simulink model "TST_CrCtl_Governor"  (R2016b)
settings: Solver=FixedStepDiscrete  StartTime=0.0  StopTime=simTime  FixedStep=sampleTime  RelTol=1e-3
values from neighbouring files (symbols this model uses):
  testCase = 1    [initTST_CrCtl_Governor_001.m]    (also in initTST_CrCtl_Governor_002.m = 2; initTST_CrCtl_Governor_003.m = 3; initTST_CrCtl_Governor_004.m = 4; initTST_CrCtl_Governor_005.m = 5)
libraries: simulink x144, UnitTest_Lib x110
(part 6 of 7)

== system TST_CrCtl_Governor/simulationInput/testSignals_R008 ==
  BC : BusCreator  Inputs=54
  spec_APP_r : FromWorkspace  VariableName=testSig_APP_r  Interpolate=off  OutputAfterFinalValue=Holding final value
  spec_AccPed_trqDes : FromWorkspace  VariableName=testSig_AccPed_trqDes  Interpolate=off  OutputAfterFinalValue=Holding final value
  spec_CoETS_trqNTCActvOff : FromWorkspace  VariableName=testSig_CoETS_trqNTCActvOff  Interpolate=off  OutputAfterFinalValue=Holding final value
  spec_CoETS_trqNTCActvOn : FromWorkspace  VariableName=testSig_CoETS_trqNTCActvOn  Interpolate=off  OutputAfterFinalValue=Holding final value
  spec_CoETS_trqUnFltLtd : FromWorkspace  VariableName=testSig_CoETS_trqUnFltLtd  Interpolate=off  OutputAfterFinalValue=Holding final value
  spec_CoVMD_trqLLim : FromWorkspace  VariableName=testSig_CoVMD_trqLLim  Interpolate=off  OutputAfterFinalValue=Holding final value
  spec_CoVeh_trqAcs : FromWorkspace  VariableName=testSig_CoVeh_trqAcs  Interpolate=off  OutputAfterFinalValue=Holding final value
  spec_CoVeh_trqPrpLimErr : FromWorkspace  VariableName=testSig_CoVeh_trqPrpLimErr  Interpolate=off  OutputAfterFinalValue=Holding final value
  spec_CrCtl_aAccThres : FromWorkspace  VariableName=testSig_CrCtl_aAccThres  Interpolate=off  OutputAfterFinalValue=Holding final value
  spec_CrCtl_aDeclThres : FromWorkspace  VariableName=testSig_CrCtl_aDeclThres  Interpolate=off  OutputAfterFinalValue=Holding final value
  spec_CrCtl_rTraV2NBeg : FromWorkspace  VariableName=testSig_CrCtl_rTraV2NBeg  Interpolate=off  OutputAfterFinalValue=Holding final value
  spec_CrCtl_st : FromWorkspace  VariableName=testSig_CrCtl_st  Interpolate=off  OutputAfterFinalValue=Holding final value
  spec_CrCtl_stGvnr : FromWorkspace  VariableName=testSig_CrCtl_stGvnr  Interpolate=off  OutputAfterFinalValue=Holding final value
  spec_CrCtl_stLck : FromWorkspace  VariableName=testSig_CrCtl_stLck  Interpolate=off  OutputAfterFinalValue=Holding final value
  spec_CrCtl_stOpFunc : FromWorkspace  VariableName=testSig_CrCtl_stOpFunc  Interpolate=off  OutputAfterFinalValue=Holding final value
  spec_CrCtl_stPtd : FromWorkspace  VariableName=testSig_CrCtl_stPtd  Interpolate=off  OutputAfterFinalValue=Holding final value
  spec_CrCtl_stReq : FromWorkspace  VariableName=testSig_CrCtl_stReq  Interpolate=off  OutputAfterFinalValue=Holding final value
  spec_CrCtl_stShOff : FromWorkspace  VariableName=testSig_CrCtl_stShOff  Interpolate=off  OutputAfterFinalValue=Holding final value
  spec_CrCtl_stSub : FromWorkspace  VariableName=testSig_CrCtl_stSub  Interpolate=off  OutputAfterFinalValue=Holding final value
  spec_CrCtl_stSubGvnr : FromWorkspace  VariableName=testSig_CrCtl_stSubGvnr  Interpolate=off  OutputAfterFinalValue=Holding final value
  spec_CrCtl_stSuspAct : FromWorkspace  VariableName=testSig_CrCtl_stSuspAct  Interpolate=off  OutputAfterFinalValue=Holding final value
  spec_CrCtl_stSuspRamp : FromWorkspace  VariableName=testSig_CrCtl_stSuspRamp  Interpolate=off  OutputAfterFinalValue=Holding final value
  spec_CrCtl_stVDirChng : FromWorkspace  VariableName=testSig_CrCtl_stVDirChng  Interpolate=off  OutputAfterFinalValue=Holding final value
  spec_CrCtl_stvHysEngBrkReq : FromWorkspace  VariableName=testSig_CrCtl_stvHysEngBrkReq  Interpolate=off  OutputAfterFinalValue=Holding final value
  spec_CrCtl_trqLead : FromWorkspace  VariableName=testSig_CrCtl_trqLead  Interpolate=off  OutputAfterFinalValue=Holding final value
  spec_CrCtl_trqLimAct : FromWorkspace  VariableName=testSig_CrCtl_trqLimAct  Interpolate=off  OutputAfterFinalValue=Holding final value
  spec_CrCtl_trqMin : FromWorkspace  VariableName=testSig_CrCtl_trqMin  Interpolate=off  OutputAfterFinalValue=Holding final value
  spec_CrCtl_trqReq : FromWorkspace  VariableName=testSig_CrCtl_trqReq  Interpolate=off  OutputAfterFinalValue=Holding final value
  spec_CrCtl_trqReqOld : FromWorkspace  VariableName=testSig_CrCtl_trqReqOld  Interpolate=off  OutputAfterFinalValue=Holding final value
  spec_CrCtl_vDes : FromWorkspace  VariableName=testSig_CrCtl_vDes  Interpolate=off  OutputAfterFinalValue=Holding final value
  spec_CrCtl_vDesAct : FromWorkspace  VariableName=testSig_CrCtl_vDesAct  Interpolate=off  OutputAfterFinalValue=Holding final value
  spec_CrCtl_vDesActOld : FromWorkspace  VariableName=testSig_CrCtl_vDesActOld  Interpolate=off  OutputAfterFinalValue=Holding final value
  spec_CrCtl_vMax : FromWorkspace  VariableName=testSig_CrCtl_vMax  Interpolate=off  OutputAfterFinalValue=Holding final value
  spec_CrCtl_vMaxDvtAcc : FromWorkspace  VariableName=testSig_CrCtl_vMaxDvtAcc  Interpolate=off  OutputAfterFinalValue=Holding final value
  spec_CrCtl_vMaxDvtDecl : FromWorkspace  VariableName=testSig_CrCtl_vMaxDvtDecl  Interpolate=off  OutputAfterFinalValue=Holding final value
  spec_CrCtl_vMin : FromWorkspace  VariableName=testSig_CrCtl_vMin  Interpolate=off  OutputAfterFinalValue=Holding final value
  spec_EBrk_stPreSelMode : FromWorkspace  VariableName=testSig_EBrk_stPreSelMode  Interpolate=off  OutputAfterFinalValue=Holding final value
  spec_EngDem_trqInrLim : FromWorkspace  VariableName=testSig_EngDem_trqInrLim  Interpolate=off  OutputAfterFinalValue=Holding final value
  spec_GlbDa_aXFlt : FromWorkspace  VariableName=testSig_GlbDa_aXFlt  Interpolate=off  OutputAfterFinalValue=Holding final value
  spec_GlbDa_vXFlt : FromWorkspace  VariableName=testSig_GlbDa_vXFlt  Interpolate=off  OutputAfterFinalValue=Holding final value
  spec_InjSys_trqLim : FromWorkspace  VariableName=testSig_InjSys_trqLim  Interpolate=off  OutputAfterFinalValue=Holding final value
  spec_PT_rTraV2N : FromWorkspace  VariableName=testSig_PT_rTraV2N  Interpolate=off  OutputAfterFinalValue=Holding final value
  spec_PT_rTrq : FromWorkspace  VariableName=testSig_PT_rTrq  Interpolate=off  OutputAfterFinalValue=Holding final value
  spec_PT_trqLos : FromWorkspace  VariableName=testSig_PT_trqLos  Interpolate=off  OutputAfterFinalValue=Holding final value
  spec_PT_trqWhl : FromWorkspace  VariableName=testSig_PT_trqWhl  Interpolate=off  OutputAfterFinalValue=Holding final value
  spec_PT_trqWhlMinEng : FromWorkspace  VariableName=testSig_PT_trqWhlMinEng  Interpolate=off  OutputAfterFinalValue=Holding final value
  spec_PT_trqWhlMinEngBrk : FromWorkspace  VariableName=testSig_PT_trqWhlMinEngBrk  Interpolate=off  OutputAfterFinalValue=Holding final value
  spec_RngMod_trqMin : FromWorkspace  VariableName=testSig_RngMod_trqMin  Interpolate=off  OutputAfterFinalValue=Holding final value
  spec_Tra_numGear : FromWorkspace  VariableName=testSig_Tra_numGear  Interpolate=off  OutputAfterFinalValue=Holding final value
  spec_VMD_trqDes : FromWorkspace  VariableName=testSig_VMD_trqDes  Interpolate=off  OutputAfterFinalValue=Holding final value
  spec_VMSAdjBtn_st : FromWorkspace  VariableName=testSig_VMSAdjBtn_st  Interpolate=off  OutputAfterFinalValue=Holding final value
  spec_VMSLmtSwt_st : FromWorkspace  VariableName=testSig_VMSLmtSwt_st  Interpolate=off  OutputAfterFinalValue=Holding final value
  spec_VehMot_rTrqDfftl : FromWorkspace  VariableName=testSig_VehMot_rTrqDfftl  Interpolate=off  OutputAfterFinalValue=Holding final value
  spec_WESDem_stCurr : FromWorkspace  VariableName=testSig_WESDem_stCurr  Interpolate=off  OutputAfterFinalValue=Holding final value
  testSignals : Outport
  wires:
  BC/1 -> testSignals/1
  spec_AccPed_trqDes/1 -> BC/1  "testSig_AccPed_trqDes"
  spec_APP_r/1 -> BC/2  "testSig_APP_r"
  spec_CoETS_trqNTCActvOff/1 -> BC/3  "testSig_CoETS_trqNTCActvOff"
  spec_CoETS_trqNTCActvOn/1 -> BC/4  "testSig_CoETS_trqNTCActvOn"
  spec_CoETS_trqUnFltLtd/1 -> BC/5  "testSig_CoETS_trqUnFltLtd"
  spec_CoVeh_trqAcs/1 -> BC/6  "testSig_CoVeh_trqAcs"
  spec_CoVeh_trqPrpLimErr/1 -> BC/7  "testSig_CoVeh_trqPrpLimErr"
  spec_CoVMD_trqLLim/1 -> BC/8  "testSig_CoVMD_trqLLim"
  spec_CrCtl_aAccThres/1 -> BC/9  "testSig_CrCtl_aAccThres"
  spec_CrCtl_aDeclThres/1 -> BC/10  "testSig_CrCtl_aDeclThres"
  spec_CrCtl_st/1 -> BC/11  "testSig_CrCtl_st"
  spec_CrCtl_stGvnr/1 -> BC/12  "testSig_CrCtl_stGvnr"
  spec_CrCtl_stLck/1 -> BC/13  "testSig_CrCtl_stLck"
  spec_CrCtl_stShOff/1 -> BC/14  "testSig_CrCtl_stShOff"
  spec_CrCtl_stSub/1 -> BC/15  "testSig_CrCtl_stSub"
  spec_CrCtl_stSubGvnr/1 -> BC/16  "testSig_CrCtl_stSubGvnr"
  spec_CrCtl_stSuspAct/1 -> BC/17  "testSig_CrCtl_stSuspAct"
  spec_CrCtl_stVDirChng/1 -> BC/18  "testSig_CrCtl_stVDirChng"
  spec_CrCtl_vDes/1 -> BC/19  "testSig_CrCtl_vDes"
  spec_CrCtl_vDesAct/1 -> BC/20  "testSig_CrCtl_vDesAct"
  spec_CrCtl_vDesActOld/1 -> BC/21  "testSig_CrCtl_vDesActOld"
  spec_CrCtl_vMaxDvtAcc/1 -> BC/22  "testSig_CrCtl_vMaxDvtAcc"
  spec_CrCtl_vMaxDvtDecl/1 -> BC/23  "testSig_CrCtl_vMaxDvtDecl"
  spec_CrCtl_vMin/1 -> BC/24  "testSig_CrCtl_vMin"
  spec_EBrk_stPreSelMode/1 -> BC/25  "testSig_EBrk_stPreSelMode"
  spec_EngDem_trqInrLim/1 -> BC/26  "testSig_EngDem_trqInrLim"
  spec_GlbDa_aXFlt/1 -> BC/27  "testSig_GlbDa_aXFlt"
  spec_GlbDa_vXFlt/1 -> BC/28  "testSig_GlbDa_vXFlt"
  spec_InjSys_trqLim/1 -> BC/29  "testSig_InjSys_trqLim"
  spec_PT_rTraV2N/1 -> BC/30  "testSig_PT_rTraV2N"
  spec_PT_rTrq/1 -> BC/31  "testSig_PT_rTrq"
  spec_PT_trqLos/1 -> BC/32  "testSig_PT_trqLos"
  spec_PT_trqWhl/1 -> BC/33  "testSig_PT_trqWhl"
  spec_PT_trqWhlMinEng/1 -> BC/34  "testSig_PT_trqWhlMinEng"
  spec_PT_trqWhlMinEngBrk/1 -> BC/35  "testSig_PT_trqWhlMinEngBrk"
  spec_RngMod_trqMin/1 -> BC/36  "testSig_RngMod_trqMin"
  spec_Tra_numGear/1 -> BC/37  "testSig_Tra_numGear"
  spec_VehMot_rTrqDfftl/1 -> BC/38  "testSig_VehMot_rTrqDfftl"
  spec_VMD_trqDes/1 -> BC/39  "testSig_VMD_trqDes"
  spec_VMSAdjBtn_st/1 -> BC/40  "testSig_VMSAdjBtn_st"
  spec_VMSLmtSwt_st/1 -> BC/41  "testSig_VMSLmtSwt_st"
  spec_WESDem_stCurr/1 -> BC/42  "testSig_WESDem_stCurr"
  spec_CrCtl_rTraV2NBeg/1 -> BC/43  "testSig_CrCtl_rTraV2NBeg"
  spec_CrCtl_stOpFunc/1 -> BC/44  "testSig_CrCtl_stOpFunc"
  spec_CrCtl_stPtd/1 -> BC/45  "testSig_CrCtl_stPtd"
  spec_CrCtl_stReq/1 -> BC/46  "testSig_CrCtl_stReq"
  spec_CrCtl_stSuspRamp/1 -> BC/47  "testSig_CrCtl_stSuspRamp"
  spec_CrCtl_stvHysEngBrkReq/1 -> BC/48  "testSig_CrCtl_stvHysEngBrkReq"
  spec_CrCtl_trqLead/1 -> BC/49  "testSig_CrCtl_trqLead"
  spec_CrCtl_trqLimAct/1 -> BC/50  "testSig_CrCtl_trqLimAct"
  spec_CrCtl_trqMin/1 -> BC/51  "testSig_CrCtl_trqMin"
  spec_CrCtl_trqReq/1 -> BC/52  "testSig_CrCtl_trqReq"
  spec_CrCtl_trqReqOld/1 -> BC/53  "testSig_CrCtl_trqReqOld"
  spec_CrCtl_vMax/1 -> BC/54  "testSig_CrCtl_vMax"

== system TST_CrCtl_Governor/simulationInput/testSignals_R009 ==
  BC : BusCreator  Inputs=54
  spec_APP_r : FromWorkspace  VariableName=testSig_APP_r  Interpolate=off  OutputAfterFinalValue=Holding final value
  spec_AccPed_trqDes : FromWorkspace  VariableName=testSig_AccPed_trqDes  Interpolate=off  OutputAfterFinalValue=Holding final value
  spec_CoETS_trqNTCActvOff : FromWorkspace  VariableName=testSig_CoETS_trqNTCActvOff  Interpolate=off  OutputAfterFinalValue=Holding final value
  spec_CoETS_trqNTCActvOn : FromWorkspace  VariableName=testSig_CoETS_trqNTCActvOn  Interpolate=off  OutputAfterFinalValue=Holding final value
  spec_CoETS_trqUnFltLtd : FromWorkspace  VariableName=testSig_CoETS_trqUnFltLtd  Interpolate=off  OutputAfterFinalValue=Holding final value
  spec_CoVMD_trqLLim : FromWorkspace  VariableName=testSig_CoVMD_trqLLim  Interpolate=off  OutputAfterFinalValue=Holding final value
  spec_CoVeh_trqAcs : FromWorkspace  VariableName=testSig_CoVeh_trqAcs  Interpolate=off  OutputAfterFinalValue=Holding final value
  spec_CoVeh_trqPrpLimErr : FromWorkspace  VariableName=testSig_CoVeh_trqPrpLimErr  Interpolate=off  OutputAfterFinalValue=Holding final value
  spec_CrCtl_aAccThres : FromWorkspace  VariableName=testSig_CrCtl_aAccThres  Interpolate=off  OutputAfterFinalValue=Holding final value
  spec_CrCtl_aDeclThres : FromWorkspace  VariableName=testSig_CrCtl_aDeclThres  Interpolate=off  OutputAfterFinalValue=Holding final value
  spec_CrCtl_rTraV2NBeg : FromWorkspace  VariableName=testSig_CrCtl_rTraV2NBeg  Interpolate=off  OutputAfterFinalValue=Holding final value
  spec_CrCtl_st : FromWorkspace  VariableName=testSig_CrCtl_st  Interpolate=off  OutputAfterFinalValue=Holding final value
  spec_CrCtl_stGvnr : FromWorkspace  VariableName=testSig_CrCtl_stGvnr  Interpolate=off  OutputAfterFinalValue=Holding final value
  spec_CrCtl_stLck : FromWorkspace  VariableName=testSig_CrCtl_stLck  Interpolate=off  OutputAfterFinalValue=Holding final value
  spec_CrCtl_stOpFunc : FromWorkspace  VariableName=testSig_CrCtl_stOpFunc  Interpolate=off  OutputAfterFinalValue=Holding final value
  spec_CrCtl_stPtd : FromWorkspace  VariableName=testSig_CrCtl_stPtd  Interpolate=off  OutputAfterFinalValue=Holding final value
  spec_CrCtl_stReq : FromWorkspace  VariableName=testSig_CrCtl_stReq  Interpolate=off  OutputAfterFinalValue=Holding final value
  spec_CrCtl_stShOff : FromWorkspace  VariableName=testSig_CrCtl_stShOff  Interpolate=off  OutputAfterFinalValue=Holding final value
  spec_CrCtl_stSub : FromWorkspace  VariableName=testSig_CrCtl_stSub  Interpolate=off  OutputAfterFinalValue=Holding final value
  spec_CrCtl_stSubGvnr : FromWorkspace  VariableName=testSig_CrCtl_stSubGvnr  Interpolate=off  OutputAfterFinalValue=Holding final value
  spec_CrCtl_stSuspAct : FromWorkspace  VariableName=testSig_CrCtl_stSuspAct  Interpolate=off  OutputAfterFinalValue=Holding final value
  spec_CrCtl_stSuspRamp : FromWorkspace  VariableName=testSig_CrCtl_stSuspRamp  Interpolate=off  OutputAfterFinalValue=Holding final value
  spec_CrCtl_stVDirChng : FromWorkspace  VariableName=testSig_CrCtl_stVDirChng  Interpolate=off  OutputAfterFinalValue=Holding final value
  spec_CrCtl_stvHysEngBrkReq : FromWorkspace  VariableName=testSig_CrCtl_stvHysEngBrkReq  Interpolate=off  OutputAfterFinalValue=Holding final value
  spec_CrCtl_trqLead : FromWorkspace  VariableName=testSig_CrCtl_trqLead  Interpolate=off  OutputAfterFinalValue=Holding final value
  spec_CrCtl_trqLimAct : FromWorkspace  VariableName=testSig_CrCtl_trqLimAct  Interpolate=off  OutputAfterFinalValue=Holding final value
  spec_CrCtl_trqMin : FromWorkspace  VariableName=testSig_CrCtl_trqMin  Interpolate=off  OutputAfterFinalValue=Holding final value
  spec_CrCtl_trqReq : FromWorkspace  VariableName=testSig_CrCtl_trqReq  Interpolate=off  OutputAfterFinalValue=Holding final value
  spec_CrCtl_trqReqOld : FromWorkspace  VariableName=testSig_CrCtl_trqReqOld  Interpolate=off  OutputAfterFinalValue=Holding final value
  spec_CrCtl_vDes : FromWorkspace  VariableName=testSig_CrCtl_vDes  Interpolate=off  OutputAfterFinalValue=Holding final value
  spec_CrCtl_vDesAct : FromWorkspace  VariableName=testSig_CrCtl_vDesAct  Interpolate=off  OutputAfterFinalValue=Holding final value
  spec_CrCtl_vDesActOld : FromWorkspace  VariableName=testSig_CrCtl_vDesActOld  Interpolate=off  OutputAfterFinalValue=Holding final value
  spec_CrCtl_vMax : FromWorkspace  VariableName=testSig_CrCtl_vMax  Interpolate=off  OutputAfterFinalValue=Holding final value
  spec_CrCtl_vMaxDvtAcc : FromWorkspace  VariableName=testSig_CrCtl_vMaxDvtAcc  Interpolate=off  OutputAfterFinalValue=Holding final value
  spec_CrCtl_vMaxDvtDecl : FromWorkspace  VariableName=testSig_CrCtl_vMaxDvtDecl  Interpolate=off  OutputAfterFinalValue=Holding final value
  spec_CrCtl_vMin : FromWorkspace  VariableName=testSig_CrCtl_vMin  Interpolate=off  OutputAfterFinalValue=Holding final value
  spec_EBrk_stPreSelMode : FromWorkspace  VariableName=testSig_EBrk_stPreSelMode  Interpolate=off  OutputAfterFinalValue=Holding final value
  spec_EngDem_trqInrLim : FromWorkspace  VariableName=testSig_EngDem_trqInrLim  Interpolate=off  OutputAfterFinalValue=Holding final value
  spec_GlbDa_aXFlt : FromWorkspace  VariableName=testSig_GlbDa_aXFlt  Interpolate=off  OutputAfterFinalValue=Holding final value
  spec_GlbDa_vXFlt : FromWorkspace  VariableName=testSig_GlbDa_vXFlt  Interpolate=off  OutputAfterFinalValue=Holding final value
  spec_InjSys_trqLim : FromWorkspace  VariableName=testSig_InjSys_trqLim  Interpolate=off  OutputAfterFinalValue=Holding final value
  spec_PT_rTraV2N : FromWorkspace  VariableName=testSig_PT_rTraV2N  Interpolate=off  OutputAfterFinalValue=Holding final value
  spec_PT_rTrq : FromWorkspace  VariableName=testSig_PT_rTrq  Interpolate=off  OutputAfterFinalValue=Holding final value
  spec_PT_trqLos : FromWorkspace  VariableName=testSig_PT_trqLos  Interpolate=off  OutputAfterFinalValue=Holding final value
  spec_PT_trqWhl : FromWorkspace  VariableName=testSig_PT_trqWhl  Interpolate=off  OutputAfterFinalValue=Holding final value
  spec_PT_trqWhlMinEng : FromWorkspace  VariableName=testSig_PT_trqWhlMinEng  Interpolate=off  OutputAfterFinalValue=Holding final value
  spec_PT_trqWhlMinEngBrk : FromWorkspace  VariableName=testSig_PT_trqWhlMinEngBrk  Interpolate=off  OutputAfterFinalValue=Holding final value
  spec_RngMod_trqMin : FromWorkspace  VariableName=testSig_RngMod_trqMin  Interpolate=off  OutputAfterFinalValue=Holding final value
  spec_Tra_numGear : FromWorkspace  VariableName=testSig_Tra_numGear  Interpolate=off  OutputAfterFinalValue=Holding final value
  spec_VMD_trqDes : FromWorkspace  VariableName=testSig_VMD_trqDes  Interpolate=off  OutputAfterFinalValue=Holding final value
  spec_VMSAdjBtn_st : FromWorkspace  VariableName=testSig_VMSAdjBtn_st  Interpolate=off  OutputAfterFinalValue=Holding final value
  spec_VMSLmtSwt_st : FromWorkspace  VariableName=testSig_VMSLmtSwt_st  Interpolate=off  OutputAfterFinalValue=Holding final value
  spec_VehMot_rTrqDfftl : FromWorkspace  VariableName=testSig_VehMot_rTrqDfftl  Interpolate=off  OutputAfterFinalValue=Holding final value
  spec_WESDem_stCurr : FromWorkspace  VariableName=testSig_WESDem_stCurr  Interpolate=off  OutputAfterFinalValue=Holding final value
  testSignals : Outport
  wires:
  BC/1 -> testSignals/1
  spec_AccPed_trqDes/1 -> BC/1  "testSig_AccPed_trqDes"
  spec_APP_r/1 -> BC/2  "testSig_APP_r"
  spec_CoETS_trqNTCActvOff/1 -> BC/3  "testSig_CoETS_trqNTCActvOff"
  spec_CoETS_trqNTCActvOn/1 -> BC/4  "testSig_CoETS_trqNTCActvOn"
  spec_CoETS_trqUnFltLtd/1 -> BC/5  "testSig_CoETS_trqUnFltLtd"
  spec_CoVeh_trqAcs/1 -> BC/6  "testSig_CoVeh_trqAcs"
  spec_CoVeh_trqPrpLimErr/1 -> BC/7  "testSig_CoVeh_trqPrpLimErr"
  spec_CoVMD_trqLLim/1 -> BC/8  "testSig_CoVMD_trqLLim"
  spec_CrCtl_aAccThres/1 -> BC/9  "testSig_CrCtl_aAccThres"
  spec_CrCtl_aDeclThres/1 -> BC/10  "testSig_CrCtl_aDeclThres"
  spec_CrCtl_st/1 -> BC/11  "testSig_CrCtl_st"
  spec_CrCtl_stGvnr/1 -> BC/12  "testSig_CrCtl_stGvnr"
  spec_CrCtl_stLck/1 -> BC/13  "testSig_CrCtl_stLck"
  spec_CrCtl_stShOff/1 -> BC/14  "testSig_CrCtl_stShOff"
  spec_CrCtl_stSub/1 -> BC/15  "testSig_CrCtl_stSub"
  spec_CrCtl_stSubGvnr/1 -> BC/16  "testSig_CrCtl_stSubGvnr"
  spec_CrCtl_stSuspAct/1 -> BC/17  "testSig_CrCtl_stSuspAct"
  spec_CrCtl_stVDirChng/1 -> BC/18  "testSig_CrCtl_stVDirChng"
  spec_CrCtl_vDes/1 -> BC/19  "testSig_CrCtl_vDes"
  spec_CrCtl_vDesAct/1 -> BC/20  "testSig_CrCtl_vDesAct"
  spec_CrCtl_vDesActOld/1 -> BC/21  "testSig_CrCtl_vDesActOld"
  spec_CrCtl_vMaxDvtAcc/1 -> BC/22  "testSig_CrCtl_vMaxDvtAcc"
  spec_CrCtl_vMaxDvtDecl/1 -> BC/23  "testSig_CrCtl_vMaxDvtDecl"
  spec_CrCtl_vMin/1 -> BC/24  "testSig_CrCtl_vMin"
  spec_EBrk_stPreSelMode/1 -> BC/25  "testSig_EBrk_stPreSelMode"
  spec_EngDem_trqInrLim/1 -> BC/26  "testSig_EngDem_trqInrLim"
  spec_GlbDa_aXFlt/1 -> BC/27  "testSig_GlbDa_aXFlt"
  spec_GlbDa_vXFlt/1 -> BC/28  "testSig_GlbDa_vXFlt"
  spec_InjSys_trqLim/1 -> BC/29  "testSig_InjSys_trqLim"
  spec_PT_rTraV2N/1 -> BC/30  "testSig_PT_rTraV2N"
  spec_PT_rTrq/1 -> BC/31  "testSig_PT_rTrq"
  spec_PT_trqLos/1 -> BC/32  "testSig_PT_trqLos"
  spec_PT_trqWhl/1 -> BC/33  "testSig_PT_trqWhl"
  spec_PT_trqWhlMinEng/1 -> BC/34  "testSig_PT_trqWhlMinEng"
  spec_PT_trqWhlMinEngBrk/1 -> BC/35  "testSig_PT_trqWhlMinEngBrk"
  spec_RngMod_trqMin/1 -> BC/36  "testSig_RngMod_trqMin"
  spec_Tra_numGear/1 -> BC/37  "testSig_Tra_numGear"
  spec_VehMot_rTrqDfftl/1 -> BC/38  "testSig_VehMot_rTrqDfftl"
  spec_VMD_trqDes/1 -> BC/39  "testSig_VMD_trqDes"
  spec_VMSAdjBtn_st/1 -> BC/40  "testSig_VMSAdjBtn_st"
  spec_VMSLmtSwt_st/1 -> BC/41  "testSig_VMSLmtSwt_st"
  spec_WESDem_stCurr/1 -> BC/42  "testSig_WESDem_stCurr"
  spec_CrCtl_rTraV2NBeg/1 -> BC/43  "testSig_CrCtl_rTraV2NBeg"
  spec_CrCtl_stOpFunc/1 -> BC/44  "testSig_CrCtl_stOpFunc"
  spec_CrCtl_stPtd/1 -> BC/45  "testSig_CrCtl_stPtd"
  spec_CrCtl_stReq/1 -> BC/46  "testSig_CrCtl_stReq"
  spec_CrCtl_stSuspRamp/1 -> BC/47  "testSig_CrCtl_stSuspRamp"
  spec_CrCtl_stvHysEngBrkReq/1 -> BC/48  "testSig_CrCtl_stvHysEngBrkReq"
  spec_CrCtl_trqLead/1 -> BC/49  "testSig_CrCtl_trqLead"
  spec_CrCtl_trqLimAct/1 -> BC/50  "testSig_CrCtl_trqLimAct"
  spec_CrCtl_trqMin/1 -> BC/51  "testSig_CrCtl_trqMin"
  spec_CrCtl_trqReq/1 -> BC/52  "testSig_CrCtl_trqReq"
  spec_CrCtl_trqReqOld/1 -> BC/53  "testSig_CrCtl_trqReqOld"
  spec_CrCtl_vMax/1 -> BC/54  "testSig_CrCtl_vMax"

== system TST_CrCtl_Governor/simulationInput/testSignals_R010 ==
  BC : BusCreator  Inputs=54
  spec_APP_r : FromWorkspace  VariableName=testSig_APP_r  Interpolate=off  OutputAfterFinalValue=Holding final value
  spec_AccPed_trqDes : FromWorkspace  VariableName=testSig_AccPed_trqDes  Interpolate=off  OutputAfterFinalValue=Holding final value
  spec_CoETS_trqNTCActvOff : FromWorkspace  VariableName=testSig_CoETS_trqNTCActvOff  Interpolate=off  OutputAfterFinalValue=Holding final value
  spec_CoETS_trqNTCActvOn : FromWorkspace  VariableName=testSig_CoETS_trqNTCActvOn  Interpolate=off  OutputAfterFinalValue=Holding final value
  spec_CoETS_trqUnFltLtd : FromWorkspace  VariableName=testSig_CoETS_trqUnFltLtd  Interpolate=off  OutputAfterFinalValue=Holding final value
  spec_CoVMD_trqLLim : FromWorkspace  VariableName=testSig_CoVMD_trqLLim  Interpolate=off  OutputAfterFinalValue=Holding final value
  spec_CoVeh_trqAcs : FromWorkspace  VariableName=testSig_CoVeh_trqAcs  Interpolate=off  OutputAfterFinalValue=Holding final value
  spec_CoVeh_trqPrpLimErr : FromWorkspace  VariableName=testSig_CoVeh_trqPrpLimErr  Interpolate=off  OutputAfterFinalValue=Holding final value
  spec_CrCtl_aAccThres : FromWorkspace  VariableName=testSig_CrCtl_aAccThres  Interpolate=off  OutputAfterFinalValue=Holding final value
  spec_CrCtl_aDeclThres : FromWorkspace  VariableName=testSig_CrCtl_aDeclThres  Interpolate=off  OutputAfterFinalValue=Holding final value
  spec_CrCtl_rTraV2NBeg : FromWorkspace  VariableName=testSig_CrCtl_rTraV2NBeg  Interpolate=off  OutputAfterFinalValue=Holding final value
  spec_CrCtl_st : FromWorkspace  VariableName=testSig_CrCtl_st  Interpolate=off  OutputAfterFinalValue=Holding final value
  spec_CrCtl_stGvnr : FromWorkspace  VariableName=testSig_CrCtl_stGvnr  Interpolate=off  OutputAfterFinalValue=Holding final value
  spec_CrCtl_stLck : FromWorkspace  VariableName=testSig_CrCtl_stLck  Interpolate=off  OutputAfterFinalValue=Holding final value
  spec_CrCtl_stOpFunc : FromWorkspace  VariableName=testSig_CrCtl_stOpFunc  Interpolate=off  OutputAfterFinalValue=Holding final value
  spec_CrCtl_stPtd : FromWorkspace  VariableName=testSig_CrCtl_stPtd  Interpolate=off  OutputAfterFinalValue=Holding final value
  spec_CrCtl_stReq : FromWorkspace  VariableName=testSig_CrCtl_stReq  Interpolate=off  OutputAfterFinalValue=Holding final value
  spec_CrCtl_stShOff : FromWorkspace  VariableName=testSig_CrCtl_stShOff  Interpolate=off  OutputAfterFinalValue=Holding final value
  spec_CrCtl_stSub : FromWorkspace  VariableName=testSig_CrCtl_stSub  Interpolate=off  OutputAfterFinalValue=Holding final value
  spec_CrCtl_stSubGvnr : FromWorkspace  VariableName=testSig_CrCtl_stSubGvnr  Interpolate=off  OutputAfterFinalValue=Holding final value
  spec_CrCtl_stSuspAct : FromWorkspace  VariableName=testSig_CrCtl_stSuspAct  Interpolate=off  OutputAfterFinalValue=Holding final value
  spec_CrCtl_stSuspRamp : FromWorkspace  VariableName=testSig_CrCtl_stSuspRamp  Interpolate=off  OutputAfterFinalValue=Holding final value
  spec_CrCtl_stVDirChng : FromWorkspace  VariableName=testSig_CrCtl_stVDirChng  Interpolate=off  OutputAfterFinalValue=Holding final value
  spec_CrCtl_stvHysEngBrkReq : FromWorkspace  VariableName=testSig_CrCtl_stvHysEngBrkReq  Interpolate=off  OutputAfterFinalValue=Holding final value
  spec_CrCtl_trqLead : FromWorkspace  VariableName=testSig_CrCtl_trqLead  Interpolate=off  OutputAfterFinalValue=Holding final value
  spec_CrCtl_trqLimAct : FromWorkspace  VariableName=testSig_CrCtl_trqLimAct  Interpolate=off  OutputAfterFinalValue=Holding final value
  spec_CrCtl_trqMin : FromWorkspace  VariableName=testSig_CrCtl_trqMin  Interpolate=off  OutputAfterFinalValue=Holding final value
  spec_CrCtl_trqReq : FromWorkspace  VariableName=testSig_CrCtl_trqReq  Interpolate=off  OutputAfterFinalValue=Holding final value
  spec_CrCtl_trqReqOld : FromWorkspace  VariableName=testSig_CrCtl_trqReqOld  Interpolate=off  OutputAfterFinalValue=Holding final value
  spec_CrCtl_vDes : FromWorkspace  VariableName=testSig_CrCtl_vDes  Interpolate=off  OutputAfterFinalValue=Holding final value
  spec_CrCtl_vDesAct : FromWorkspace  VariableName=testSig_CrCtl_vDesAct  Interpolate=off  OutputAfterFinalValue=Holding final value
  spec_CrCtl_vDesActOld : FromWorkspace  VariableName=testSig_CrCtl_vDesActOld  Interpolate=off  OutputAfterFinalValue=Holding final value
  spec_CrCtl_vMax : FromWorkspace  VariableName=testSig_CrCtl_vMax  Interpolate=off  OutputAfterFinalValue=Holding final value
  spec_CrCtl_vMaxDvtAcc : FromWorkspace  VariableName=testSig_CrCtl_vMaxDvtAcc  Interpolate=off  OutputAfterFinalValue=Holding final value
  spec_CrCtl_vMaxDvtDecl : FromWorkspace  VariableName=testSig_CrCtl_vMaxDvtDecl  Interpolate=off  OutputAfterFinalValue=Holding final value
  spec_CrCtl_vMin : FromWorkspace  VariableName=testSig_CrCtl_vMin  Interpolate=off  OutputAfterFinalValue=Holding final value
  spec_EBrk_stPreSelMode : FromWorkspace  VariableName=testSig_EBrk_stPreSelMode  Interpolate=off  OutputAfterFinalValue=Holding final value
  spec_EngDem_trqInrLim : FromWorkspace  VariableName=testSig_EngDem_trqInrLim  Interpolate=off  OutputAfterFinalValue=Holding final value
  spec_GlbDa_aXFlt : FromWorkspace  VariableName=testSig_GlbDa_aXFlt  Interpolate=off  OutputAfterFinalValue=Holding final value
  spec_GlbDa_vXFlt : FromWorkspace  VariableName=testSig_GlbDa_vXFlt  Interpolate=off  OutputAfterFinalValue=Holding final value
  spec_InjSys_trqLim : FromWorkspace  VariableName=testSig_InjSys_trqLim  Interpolate=off  OutputAfterFinalValue=Holding final value
  spec_PT_rTraV2N : FromWorkspace  VariableName=testSig_PT_rTraV2N  Interpolate=off  OutputAfterFinalValue=Holding final value
  spec_PT_rTrq : FromWorkspace  VariableName=testSig_PT_rTrq  Interpolate=off  OutputAfterFinalValue=Holding final value
  spec_PT_trqLos : FromWorkspace  VariableName=testSig_PT_trqLos  Interpolate=off  OutputAfterFinalValue=Holding final value
  spec_PT_trqWhl : FromWorkspace  VariableName=testSig_PT_trqWhl  Interpolate=off  OutputAfterFinalValue=Holding final value
  spec_PT_trqWhlMinEng : FromWorkspace  VariableName=testSig_PT_trqWhlMinEng  Interpolate=off  OutputAfterFinalValue=Holding final value
  spec_PT_trqWhlMinEngBrk : FromWorkspace  VariableName=testSig_PT_trqWhlMinEngBrk  Interpolate=off  OutputAfterFinalValue=Holding final value
  spec_RngMod_trqMin : FromWorkspace  VariableName=testSig_RngMod_trqMin  Interpolate=off  OutputAfterFinalValue=Holding final value
  spec_Tra_numGear : FromWorkspace  VariableName=testSig_Tra_numGear  Interpolate=off  OutputAfterFinalValue=Holding final value
  spec_VMD_trqDes : FromWorkspace  VariableName=testSig_VMD_trqDes  Interpolate=off  OutputAfterFinalValue=Holding final value
  spec_VMSAdjBtn_st : FromWorkspace  VariableName=testSig_VMSAdjBtn_st  Interpolate=off  OutputAfterFinalValue=Holding final value
  spec_VMSLmtSwt_st : FromWorkspace  VariableName=testSig_VMSLmtSwt_st  Interpolate=off  OutputAfterFinalValue=Holding final value
  spec_VehMot_rTrqDfftl : FromWorkspace  VariableName=testSig_VehMot_rTrqDfftl  Interpolate=off  OutputAfterFinalValue=Holding final value
  spec_WESDem_stCurr : FromWorkspace  VariableName=testSig_WESDem_stCurr  Interpolate=off  OutputAfterFinalValue=Holding final value
  testSignals : Outport
  wires:
  BC/1 -> testSignals/1
  spec_AccPed_trqDes/1 -> BC/1  "testSig_AccPed_trqDes"
  spec_APP_r/1 -> BC/2  "testSig_APP_r"
  spec_CoETS_trqNTCActvOff/1 -> BC/3  "testSig_CoETS_trqNTCActvOff"
  spec_CoETS_trqNTCActvOn/1 -> BC/4  "testSig_CoETS_trqNTCActvOn"
  spec_CoETS_trqUnFltLtd/1 -> BC/5  "testSig_CoETS_trqUnFltLtd"
  spec_CoVeh_trqAcs/1 -> BC/6  "testSig_CoVeh_trqAcs"
  spec_CoVeh_trqPrpLimErr/1 -> BC/7  "testSig_CoVeh_trqPrpLimErr"
  spec_CoVMD_trqLLim/1 -> BC/8  "testSig_CoVMD_trqLLim"
  spec_CrCtl_aAccThres/1 -> BC/9  "testSig_CrCtl_aAccThres"
  spec_CrCtl_aDeclThres/1 -> BC/10  "testSig_CrCtl_aDeclThres"
  spec_CrCtl_st/1 -> BC/11  "testSig_CrCtl_st"
  spec_CrCtl_stGvnr/1 -> BC/12  "testSig_CrCtl_stGvnr"
  spec_CrCtl_stLck/1 -> BC/13  "testSig_CrCtl_stLck"
  spec_CrCtl_stShOff/1 -> BC/14  "testSig_CrCtl_stShOff"
  spec_CrCtl_stSub/1 -> BC/15  "testSig_CrCtl_stSub"
  spec_CrCtl_stSubGvnr/1 -> BC/16  "testSig_CrCtl_stSubGvnr"
  spec_CrCtl_stSuspAct/1 -> BC/17  "testSig_CrCtl_stSuspAct"
  spec_CrCtl_stVDirChng/1 -> BC/18  "testSig_CrCtl_stVDirChng"
  spec_CrCtl_vDes/1 -> BC/19  "testSig_CrCtl_vDes"
  spec_CrCtl_vDesAct/1 -> BC/20  "testSig_CrCtl_vDesAct"
  spec_CrCtl_vDesActOld/1 -> BC/21  "testSig_CrCtl_vDesActOld"
  spec_CrCtl_vMaxDvtAcc/1 -> BC/22  "testSig_CrCtl_vMaxDvtAcc"
  spec_CrCtl_vMaxDvtDecl/1 -> BC/23  "testSig_CrCtl_vMaxDvtDecl"
  spec_CrCtl_vMin/1 -> BC/24  "testSig_CrCtl_vMin"
  spec_EBrk_stPreSelMode/1 -> BC/25  "testSig_EBrk_stPreSelMode"
  spec_EngDem_trqInrLim/1 -> BC/26  "testSig_EngDem_trqInrLim"
  spec_GlbDa_aXFlt/1 -> BC/27  "testSig_GlbDa_aXFlt"
  spec_GlbDa_vXFlt/1 -> BC/28  "testSig_GlbDa_vXFlt"
  spec_InjSys_trqLim/1 -> BC/29  "testSig_InjSys_trqLim"
  spec_PT_rTraV2N/1 -> BC/30  "testSig_PT_rTraV2N"
  spec_PT_rTrq/1 -> BC/31  "testSig_PT_rTrq"
  spec_PT_trqLos/1 -> BC/32  "testSig_PT_trqLos"
  spec_PT_trqWhl/1 -> BC/33  "testSig_PT_trqWhl"
  spec_PT_trqWhlMinEng/1 -> BC/34  "testSig_PT_trqWhlMinEng"
  spec_PT_trqWhlMinEngBrk/1 -> BC/35  "testSig_PT_trqWhlMinEngBrk"
  spec_RngMod_trqMin/1 -> BC/36  "testSig_RngMod_trqMin"
  spec_Tra_numGear/1 -> BC/37  "testSig_Tra_numGear"
  spec_VehMot_rTrqDfftl/1 -> BC/38  "testSig_VehMot_rTrqDfftl"
  spec_VMD_trqDes/1 -> BC/39  "testSig_VMD_trqDes"
  spec_VMSAdjBtn_st/1 -> BC/40  "testSig_VMSAdjBtn_st"
  spec_VMSLmtSwt_st/1 -> BC/41  "testSig_VMSLmtSwt_st"
  spec_WESDem_stCurr/1 -> BC/42  "testSig_WESDem_stCurr"
  spec_CrCtl_rTraV2NBeg/1 -> BC/43  "testSig_CrCtl_rTraV2NBeg"
  spec_CrCtl_stOpFunc/1 -> BC/44  "testSig_CrCtl_stOpFunc"
  spec_CrCtl_stPtd/1 -> BC/45  "testSig_CrCtl_stPtd"
  spec_CrCtl_stReq/1 -> BC/46  "testSig_CrCtl_stReq"
  spec_CrCtl_stSuspRamp/1 -> BC/47  "testSig_CrCtl_stSuspRamp"
  spec_CrCtl_stvHysEngBrkReq/1 -> BC/48  "testSig_CrCtl_stvHysEngBrkReq"
  spec_CrCtl_trqLead/1 -> BC/49  "testSig_CrCtl_trqLead"
  spec_CrCtl_trqLimAct/1 -> BC/50  "testSig_CrCtl_trqLimAct"
  spec_CrCtl_trqMin/1 -> BC/51  "testSig_CrCtl_trqMin"
  spec_CrCtl_trqReq/1 -> BC/52  "testSig_CrCtl_trqReq"
  spec_CrCtl_trqReqOld/1 -> BC/53  "testSig_CrCtl_trqReqOld"
  spec_CrCtl_vMax/1 -> BC/54  "testSig_CrCtl_vMax"

== system TST_CrCtl_Governor/simulationInput/testSignals_R011 ==
  BC : BusCreator  Inputs=54
  spec_APP_r : FromWorkspace  VariableName=testSig_APP_r  Interpolate=off  OutputAfterFinalValue=Holding final value
  spec_AccPed_trqDes : FromWorkspace  VariableName=testSig_AccPed_trqDes  Interpolate=off  OutputAfterFinalValue=Holding final value
  spec_CoETS_trqNTCActvOff : FromWorkspace  VariableName=testSig_CoETS_trqNTCActvOff  Interpolate=off  OutputAfterFinalValue=Holding final value
  spec_CoETS_trqNTCActvOn : FromWorkspace  VariableName=testSig_CoETS_trqNTCActvOn  Interpolate=off  OutputAfterFinalValue=Holding final value
  spec_CoETS_trqUnFltLtd : FromWorkspace  VariableName=testSig_CoETS_trqUnFltLtd  Interpolate=off  OutputAfterFinalValue=Holding final value
  spec_CoVMD_trqLLim : FromWorkspace  VariableName=testSig_CoVMD_trqLLim  Interpolate=off  OutputAfterFinalValue=Holding final value
  spec_CoVeh_trqAcs : FromWorkspace  VariableName=testSig_CoVeh_trqAcs  Interpolate=off  OutputAfterFinalValue=Holding final value
  spec_CoVeh_trqPrpLimErr : FromWorkspace  VariableName=testSig_CoVeh_trqPrpLimErr  Interpolate=off  OutputAfterFinalValue=Holding final value
  spec_CrCtl_aAccThres : FromWorkspace  VariableName=testSig_CrCtl_aAccThres  Interpolate=off  OutputAfterFinalValue=Holding final value
  spec_CrCtl_aDeclThres : FromWorkspace  VariableName=testSig_CrCtl_aDeclThres  Interpolate=off  OutputAfterFinalValue=Holding final value
  spec_CrCtl_rTraV2NBeg : FromWorkspace  VariableName=testSig_CrCtl_rTraV2NBeg  Interpolate=off  OutputAfterFinalValue=Holding final value
  spec_CrCtl_st : FromWorkspace  VariableName=testSig_CrCtl_st  Interpolate=off  OutputAfterFinalValue=Holding final value
  spec_CrCtl_stGvnr : FromWorkspace  VariableName=testSig_CrCtl_stGvnr  Interpolate=off  OutputAfterFinalValue=Holding final value
  spec_CrCtl_stLck : FromWorkspace  VariableName=testSig_CrCtl_stLck  Interpolate=off  OutputAfterFinalValue=Holding final value
  spec_CrCtl_stOpFunc : FromWorkspace  VariableName=testSig_CrCtl_stOpFunc  Interpolate=off  OutputAfterFinalValue=Holding final value
  spec_CrCtl_stPtd : FromWorkspace  VariableName=testSig_CrCtl_stPtd  Interpolate=off  OutputAfterFinalValue=Holding final value
  spec_CrCtl_stReq : FromWorkspace  VariableName=testSig_CrCtl_stReq  Interpolate=off  OutputAfterFinalValue=Holding final value
  spec_CrCtl_stShOff : FromWorkspace  VariableName=testSig_CrCtl_stShOff  Interpolate=off  OutputAfterFinalValue=Holding final value
  spec_CrCtl_stSub : FromWorkspace  VariableName=testSig_CrCtl_stSub  Interpolate=off  OutputAfterFinalValue=Holding final value
  spec_CrCtl_stSubGvnr : FromWorkspace  VariableName=testSig_CrCtl_stSubGvnr  Interpolate=off  OutputAfterFinalValue=Holding final value
  spec_CrCtl_stSuspAct : FromWorkspace  VariableName=testSig_CrCtl_stSuspAct  Interpolate=off  OutputAfterFinalValue=Holding final value
  spec_CrCtl_stSuspRamp : FromWorkspace  VariableName=testSig_CrCtl_stSuspRamp  Interpolate=off  OutputAfterFinalValue=Holding final value
  spec_CrCtl_stVDirChng : FromWorkspace  VariableName=testSig_CrCtl_stVDirChng  Interpolate=off  OutputAfterFinalValue=Holding final value
  spec_CrCtl_stvHysEngBrkReq : FromWorkspace  VariableName=testSig_CrCtl_stvHysEngBrkReq  Interpolate=off  OutputAfterFinalValue=Holding final value
  spec_CrCtl_trqLead : FromWorkspace  VariableName=testSig_CrCtl_trqLead  Interpolate=off  OutputAfterFinalValue=Holding final value
  spec_CrCtl_trqLimAct : FromWorkspace  VariableName=testSig_CrCtl_trqLimAct  Interpolate=off  OutputAfterFinalValue=Holding final value
  spec_CrCtl_trqMin : FromWorkspace  VariableName=testSig_CrCtl_trqMin  Interpolate=off  OutputAfterFinalValue=Holding final value
  spec_CrCtl_trqReq : FromWorkspace  VariableName=testSig_CrCtl_trqReq  Interpolate=off  OutputAfterFinalValue=Holding final value
  spec_CrCtl_trqReqOld : FromWorkspace  VariableName=testSig_CrCtl_trqReqOld  Interpolate=off  OutputAfterFinalValue=Holding final value
  spec_CrCtl_vDes : FromWorkspace  VariableName=testSig_CrCtl_vDes  Interpolate=off  OutputAfterFinalValue=Holding final value
  spec_CrCtl_vDesAct : FromWorkspace  VariableName=testSig_CrCtl_vDesAct  Interpolate=off  OutputAfterFinalValue=Holding final value
  spec_CrCtl_vDesActOld : FromWorkspace  VariableName=testSig_CrCtl_vDesActOld  Interpolate=off  OutputAfterFinalValue=Holding final value
  spec_CrCtl_vMax : FromWorkspace  VariableName=testSig_CrCtl_vMax  Interpolate=off  OutputAfterFinalValue=Holding final value
  spec_CrCtl_vMaxDvtAcc : FromWorkspace  VariableName=testSig_CrCtl_vMaxDvtAcc  Interpolate=off  OutputAfterFinalValue=Holding final value
  spec_CrCtl_vMaxDvtDecl : FromWorkspace  VariableName=testSig_CrCtl_vMaxDvtDecl  Interpolate=off  OutputAfterFinalValue=Holding final value
  spec_CrCtl_vMin : FromWorkspace  VariableName=testSig_CrCtl_vMin  Interpolate=off  OutputAfterFinalValue=Holding final value
  spec_EBrk_stPreSelMode : FromWorkspace  VariableName=testSig_EBrk_stPreSelMode  Interpolate=off  OutputAfterFinalValue=Holding final value
  spec_EngDem_trqInrLim : FromWorkspace  VariableName=testSig_EngDem_trqInrLim  Interpolate=off  OutputAfterFinalValue=Holding final value
  spec_GlbDa_aXFlt : FromWorkspace  VariableName=testSig_GlbDa_aXFlt  Interpolate=off  OutputAfterFinalValue=Holding final value
  spec_GlbDa_vXFlt : FromWorkspace  VariableName=testSig_GlbDa_vXFlt  Interpolate=off  OutputAfterFinalValue=Holding final value
  spec_InjSys_trqLim : FromWorkspace  VariableName=testSig_InjSys_trqLim  Interpolate=off  OutputAfterFinalValue=Holding final value
  spec_PT_rTraV2N : FromWorkspace  VariableName=testSig_PT_rTraV2N  Interpolate=off  OutputAfterFinalValue=Holding final value
  spec_PT_rTrq : FromWorkspace  VariableName=testSig_PT_rTrq  Interpolate=off  OutputAfterFinalValue=Holding final value
  spec_PT_trqLos : FromWorkspace  VariableName=testSig_PT_trqLos  Interpolate=off  OutputAfterFinalValue=Holding final value
  spec_PT_trqWhl : FromWorkspace  VariableName=testSig_PT_trqWhl  Interpolate=off  OutputAfterFinalValue=Holding final value
  spec_PT_trqWhlMinEng : FromWorkspace  VariableName=testSig_PT_trqWhlMinEng  Interpolate=off  OutputAfterFinalValue=Holding final value
  spec_PT_trqWhlMinEngBrk : FromWorkspace  VariableName=testSig_PT_trqWhlMinEngBrk  Interpolate=off  OutputAfterFinalValue=Holding final value
  spec_RngMod_trqMin : FromWorkspace  VariableName=testSig_RngMod_trqMin  Interpolate=off  OutputAfterFinalValue=Holding final value
  spec_Tra_numGear : FromWorkspace  VariableName=testSig_Tra_numGear  Interpolate=off  OutputAfterFinalValue=Holding final value
  spec_VMD_trqDes : FromWorkspace  VariableName=testSig_VMD_trqDes  Interpolate=off  OutputAfterFinalValue=Holding final value
  spec_VMSAdjBtn_st : FromWorkspace  VariableName=testSig_VMSAdjBtn_st  Interpolate=off  OutputAfterFinalValue=Holding final value
  spec_VMSLmtSwt_st : FromWorkspace  VariableName=testSig_VMSLmtSwt_st  Interpolate=off  OutputAfterFinalValue=Holding final value
  spec_VehMot_rTrqDfftl : FromWorkspace  VariableName=testSig_VehMot_rTrqDfftl  Interpolate=off  OutputAfterFinalValue=Holding final value
  spec_WESDem_stCurr : FromWorkspace  VariableName=testSig_WESDem_stCurr  Interpolate=off  OutputAfterFinalValue=Holding final value
  testSignals : Outport
  wires:
  BC/1 -> testSignals/1
  spec_AccPed_trqDes/1 -> BC/1  "testSig_AccPed_trqDes"
  spec_APP_r/1 -> BC/2  "testSig_APP_r"
  spec_CoETS_trqNTCActvOff/1 -> BC/3  "testSig_CoETS_trqNTCActvOff"
  spec_CoETS_trqNTCActvOn/1 -> BC/4  "testSig_CoETS_trqNTCActvOn"
  spec_CoETS_trqUnFltLtd/1 -> BC/5  "testSig_CoETS_trqUnFltLtd"
  spec_CoVeh_trqAcs/1 -> BC/6  "testSig_CoVeh_trqAcs"
  spec_CoVeh_trqPrpLimErr/1 -> BC/7  "testSig_CoVeh_trqPrpLimErr"
  spec_CoVMD_trqLLim/1 -> BC/8  "testSig_CoVMD_trqLLim"
  spec_CrCtl_aAccThres/1 -> BC/9  "testSig_CrCtl_aAccThres"
  spec_CrCtl_aDeclThres/1 -> BC/10  "testSig_CrCtl_aDeclThres"
  spec_CrCtl_st/1 -> BC/11  "testSig_CrCtl_st"
  spec_CrCtl_stGvnr/1 -> BC/12  "testSig_CrCtl_stGvnr"
  spec_CrCtl_stLck/1 -> BC/13  "testSig_CrCtl_stLck"
  spec_CrCtl_stShOff/1 -> BC/14  "testSig_CrCtl_stShOff"
  spec_CrCtl_stSub/1 -> BC/15  "testSig_CrCtl_stSub"
  spec_CrCtl_stSubGvnr/1 -> BC/16  "testSig_CrCtl_stSubGvnr"
  spec_CrCtl_stSuspAct/1 -> BC/17  "testSig_CrCtl_stSuspAct"
  spec_CrCtl_stVDirChng/1 -> BC/18  "testSig_CrCtl_stVDirChng"
  spec_CrCtl_vDes/1 -> BC/19  "testSig_CrCtl_vDes"
  spec_CrCtl_vDesAct/1 -> BC/20  "testSig_CrCtl_vDesAct"
  spec_CrCtl_vDesActOld/1 -> BC/21  "testSig_CrCtl_vDesActOld"
  spec_CrCtl_vMaxDvtAcc/1 -> BC/22  "testSig_CrCtl_vMaxDvtAcc"
  spec_CrCtl_vMaxDvtDecl/1 -> BC/23  "testSig_CrCtl_vMaxDvtDecl"
  spec_CrCtl_vMin/1 -> BC/24  "testSig_CrCtl_vMin"
  spec_EBrk_stPreSelMode/1 -> BC/25  "testSig_EBrk_stPreSelMode"
  spec_EngDem_trqInrLim/1 -> BC/26  "testSig_EngDem_trqInrLim"
  spec_GlbDa_aXFlt/1 -> BC/27  "testSig_GlbDa_aXFlt"
  spec_GlbDa_vXFlt/1 -> BC/28  "testSig_GlbDa_vXFlt"
  spec_InjSys_trqLim/1 -> BC/29  "testSig_InjSys_trqLim"
  spec_PT_rTraV2N/1 -> BC/30  "testSig_PT_rTraV2N"
  spec_PT_rTrq/1 -> BC/31  "testSig_PT_rTrq"
  spec_PT_trqLos/1 -> BC/32  "testSig_PT_trqLos"
  spec_PT_trqWhl/1 -> BC/33  "testSig_PT_trqWhl"
  spec_PT_trqWhlMinEng/1 -> BC/34  "testSig_PT_trqWhlMinEng"
  spec_PT_trqWhlMinEngBrk/1 -> BC/35  "testSig_PT_trqWhlMinEngBrk"
  spec_RngMod_trqMin/1 -> BC/36  "testSig_RngMod_trqMin"
  spec_Tra_numGear/1 -> BC/37  "testSig_Tra_numGear"
  spec_VehMot_rTrqDfftl/1 -> BC/38  "testSig_VehMot_rTrqDfftl"
  spec_VMD_trqDes/1 -> BC/39  "testSig_VMD_trqDes"
  spec_VMSAdjBtn_st/1 -> BC/40  "testSig_VMSAdjBtn_st"
  spec_VMSLmtSwt_st/1 -> BC/41  "testSig_VMSLmtSwt_st"
  spec_WESDem_stCurr/1 -> BC/42  "testSig_WESDem_stCurr"
  spec_CrCtl_rTraV2NBeg/1 -> BC/43  "testSig_CrCtl_rTraV2NBeg"
  spec_CrCtl_stOpFunc/1 -> BC/44  "testSig_CrCtl_stOpFunc"
  spec_CrCtl_stPtd/1 -> BC/45  "testSig_CrCtl_stPtd"
  spec_CrCtl_stReq/1 -> BC/46  "testSig_CrCtl_stReq"
  spec_CrCtl_stSuspRamp/1 -> BC/47  "testSig_CrCtl_stSuspRamp"
  spec_CrCtl_stvHysEngBrkReq/1 -> BC/48  "testSig_CrCtl_stvHysEngBrkReq"
  spec_CrCtl_trqLead/1 -> BC/49  "testSig_CrCtl_trqLead"
  spec_CrCtl_trqLimAct/1 -> BC/50  "testSig_CrCtl_trqLimAct"
  spec_CrCtl_trqMin/1 -> BC/51  "testSig_CrCtl_trqMin"
  spec_CrCtl_trqReq/1 -> BC/52  "testSig_CrCtl_trqReq"
  spec_CrCtl_trqReqOld/1 -> BC/53  "testSig_CrCtl_trqReqOld"
  spec_CrCtl_vMax/1 -> BC/54  "testSig_CrCtl_vMax"

== system TST_CrCtl_Governor/compareSignals/Requirement_001/specifyOutputs ==
  sig_Req_Bus : Inport
  sig_Result_Bus : Inport  Port=2
  AndN : Logic  Inputs=12
  BS_Req : BusSelector  OutputSignals=testSig_CrCtl_rTraV2NBeg,testSig_CrCtl_stOpFunc,testSig_CrCtl_stPtd,testSig_CrCtl_stReq,testSig_CrCtl_stSuspRamp,testSig_CrCtl_stvHysEngBrkReq,testSig_CrCtl_trqLead,testSig_CrCtl_trqLimAct,testSig_CrCtl_trqMin,testSig_CrCtl_trqReq,testSig_CrCtl_trqReqOld,testSig_CrCtl_vMax
  BS_Result : BusSelector  OutputSignals=CrCtl_rTraV2NBeg,CrCtl_stOpFunc,CrCtl_stPtd,CrCtl_stReq,CrCtl_stSuspRamp,CrCtl_stvHysEngBrkReq,CrCtl_trqLead,CrCtl_trqLimAct,CrCtl_trqMin,CrCtl_trqReq,CrCtl_trqReqOld,CrCtl_vMax
  Bitwise_And{1..12} (12 alike) : simulink/Logic and Bit Operations/Bitwise Operator  logicop=AND  UseBitMask=off  BitMask=bin2dec('11011001')  BitMaskRealWorld=Stored Integer
  Relational Operator : RelationalOperator  Operator===  OutDataTypeStr=boolean  RndMeth=Simplest
  Relational Operator1 : RelationalOperator  Operator===  OutDataTypeStr=boolean  RndMeth=Simplest
  Scope : Scope  NumInputPorts=12
  Scope{1..12} (12 alike) : Scope  NumInputPorts=2
  cmp_{1,3..4,6..12} (10 alike) : UnitTest_Lib/RoughlyEqual  slope=0.1
  result_tws : ToWorkspace  VariableName=spec_result_001
  tws_1 : ToWorkspace  VariableName=spec_req_001_001
  tws_10 : ToWorkspace  VariableName=spec_req_001_010
  tws_11 : ToWorkspace  VariableName=spec_req_001_011
  tws_12 : ToWorkspace  VariableName=spec_req_001_012
  tws_2 : ToWorkspace  VariableName=spec_req_001_002
  tws_3 : ToWorkspace  VariableName=spec_req_001_003
  tws_4 : ToWorkspace  VariableName=spec_req_001_004
  tws_5 : ToWorkspace  VariableName=spec_req_001_005
  tws_6 : ToWorkspace  VariableName=spec_req_001_006
  tws_7 : ToWorkspace  VariableName=spec_req_001_007
  tws_8 : ToWorkspace  VariableName=spec_req_001_008
  tws_9 : ToWorkspace  VariableName=spec_req_001_009
  result : Outport
  wires:
  sig_Req_Bus/1 -> BS_Req/1
  sig_Result_Bus/1 -> BS_Result/1
  AndN/1 -> result/1, result_tws/1
  BS_Req/1 -> cmp_1/1, Scope1/1  "<testSig_CrCtl_rTraV2NBeg>"
  BS_Result/1 -> cmp_1/2, Scope1/2  "<CrCtl_rTraV2NBeg>"
  cmp_1/1 -> Bitwise_And1/1
  Bitwise_And1/1 -> AndN/1, Scope/1, tws_1/1
  BS_Req/2 -> Relational Operator/1, Scope2/1  "<testSig_CrCtl_stOpFunc>"
  BS_Result/2 -> Scope2/2, Relational Operator/2  "<CrCtl_stOpFunc>"
  Relational Operator/1 -> Bitwise_And2/1
  Bitwise_And2/1 -> AndN/2, Scope/2, tws_2/1
  BS_Req/3 -> cmp_3/1, Scope3/1  "<testSig_CrCtl_stPtd>"
  BS_Result/3 -> cmp_3/2, Scope3/2  "<CrCtl_stPtd>"
  cmp_3/1 -> Bitwise_And3/1
  Bitwise_And3/1 -> AndN/3, Scope/3, tws_3/1
  BS_Req/4 -> cmp_4/1, Scope4/1  "<testSig_CrCtl_stReq>"
  BS_Result/4 -> cmp_4/2, Scope4/2  "<CrCtl_stReq>"
  cmp_4/1 -> Bitwise_And4/1
  Bitwise_And4/1 -> AndN/4, Scope/4, tws_4/1
  BS_Req/5 -> Relational Operator1/1, Scope5/1  "<testSig_CrCtl_stSuspRamp>"
  BS_Result/5 -> Scope5/2, Relational Operator1/2  "<CrCtl_stSuspRamp>"
  Relational Operator1/1 -> Bitwise_And5/1
  Bitwise_And5/1 -> AndN/5, Scope/5, tws_5/1
  BS_Req/6 -> cmp_6/1, Scope6/1  "<testSig_CrCtl_stvHysEngBrkReq>"
  BS_Result/6 -> cmp_6/2, Scope6/2  "<CrCtl_stvHysEngBrkReq>"
  cmp_6/1 -> Bitwise_And6/1
  Bitwise_And6/1 -> AndN/6, Scope/6, tws_6/1
  BS_Req/7 -> cmp_7/1, Scope7/1  "<testSig_CrCtl_trqLead>"
  BS_Result/7 -> cmp_7/2, Scope7/2  "<CrCtl_trqLead>"
  cmp_7/1 -> Bitwise_And7/1
  Bitwise_And7/1 -> AndN/7, Scope/7, tws_7/1
  BS_Req/8 -> cmp_8/1, Scope8/1  "<testSig_CrCtl_trqLimAct>"
  BS_Result/8 -> cmp_8/2, Scope8/2  "<CrCtl_trqLimAct>"
  cmp_8/1 -> Bitwise_And8/1
  Bitwise_And8/1 -> AndN/8, Scope/8, tws_8/1
  BS_Req/9 -> cmp_9/1, Scope9/1  "<testSig_CrCtl_trqMin>"
  BS_Result/9 -> cmp_9/2, Scope9/2  "<CrCtl_trqMin>"
  cmp_9/1 -> Bitwise_And9/1
  Bitwise_And9/1 -> AndN/9, Scope/9, tws_9/1
  BS_Req/10 -> cmp_10/1, Scope10/1  "<testSig_CrCtl_trqReq>"
  BS_Result/10 -> cmp_10/2, Scope10/2  "<CrCtl_trqReq>"
  cmp_10/1 -> Bitwise_And10/1
  Bitwise_And10/1 -> AndN/10, Scope/10, tws_10/1
  BS_Req/11 -> cmp_11/1, Scope11/1  "<testSig_CrCtl_trqReqOld>"
  BS_Result/11 -> cmp_11/2, Scope11/2  "<CrCtl_trqReqOld>"
  cmp_11/1 -> Bitwise_And11/1
  Bitwise_And11/1 -> AndN/11, Scope/11, tws_11/1
  BS_Req/12 -> cmp_12/1, Scope12/1  "<testSig_CrCtl_vMax>"
  BS_Result/12 -> cmp_12/2, Scope12/2  "<CrCtl_vMax>"
  cmp_12/1 -> Bitwise_And12/1
  Bitwise_And12/1 -> AndN/12, Scope/12, tws_12/1
